simulink model "untitled1"  (R2023b)
settings: Solver=VariableStepAuto  StartTime=0.0  StopTime=10.0  RelTol=1e-3
libraries: dspsigops x1
settings Model: Creator=a2  LastModifiedBy=a2

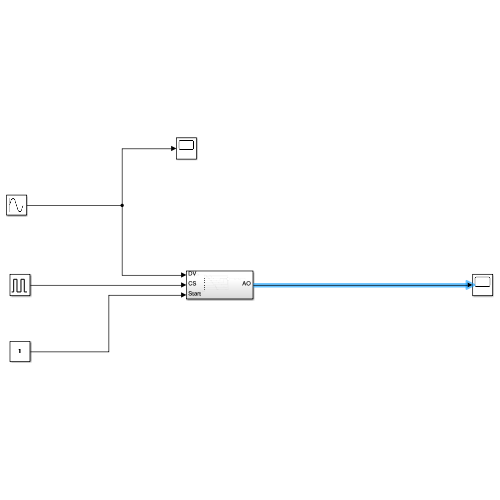
[thumbnail: Simulink's stored preview of the top-level diagram]
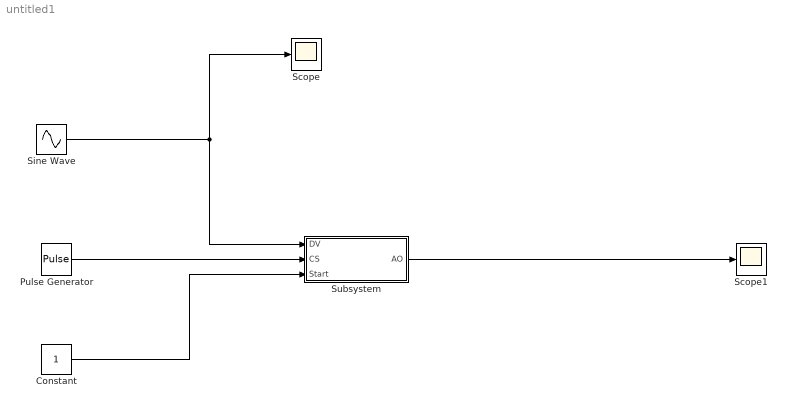
== system untitled1 ==
  Constant : Constant
  Pulse Generator : DiscretePulseGenerator  PulseType=Time based  Period=10  PulseWidth=5
  Scope : Scope
  Scope1 : Scope
  Sine Wave : Sin  SampleTime=0
  Subsystem : Subsystem
  wires:
  Sine Wave/1 -> Subsystem/1(DV), Scope/1
  Pulse Generator/1 -> Subsystem/2(CS)
  Constant/1 -> Subsystem/3(Start)
  Subsystem/1(AO) -> Scope1/1

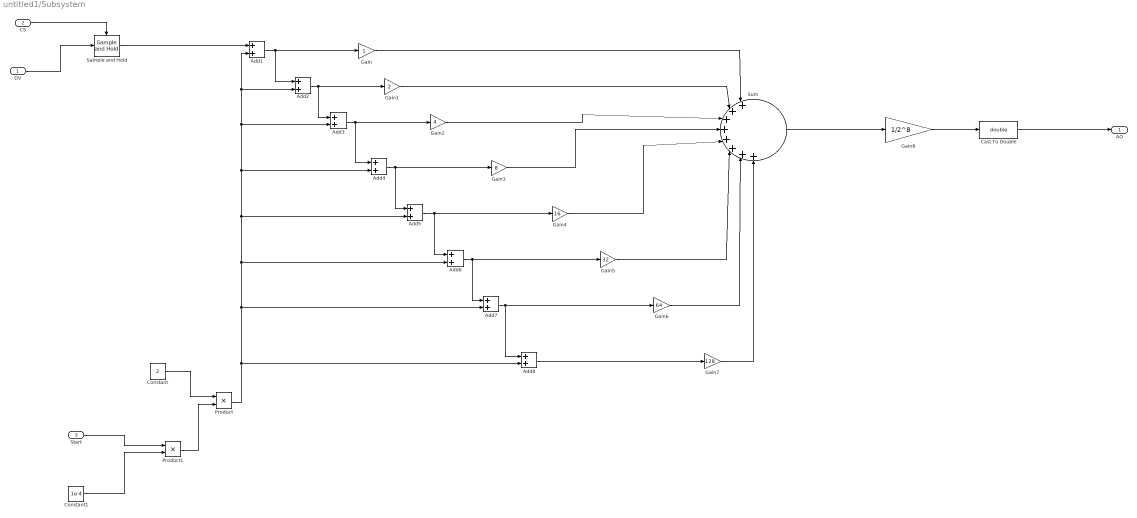
== system untitled1/Subsystem ==
  DV : Inport
  CS : Inport  Port=2
  Start : Inport  Port=3
  Add{1..8} (8 alike) : Sum
  Cast To Double : DataTypeConversion  OutDataTypeStr=double  SaturateOnIntegerOverflow=off  RndMeth=Floor
  Constant : Constant  Value=2
  Constant1 : Constant  Value=1e-4
  Gain : Gain
  Gain1 : Gain  Gain=2
  Gain2 : Gain  Gain=4
  Gain3 : Gain  Gain=8
  Gain4 : Gain  Gain=16
  Gain5 : Gain  Gain=32
  Gain6 : Gain  Gain=64
  Gain7 : Gain  Gain=128
  Gain8 : Gain  Gain=1/2^8
  Product : Product
  Product1 : Product
  Sample and Hold : dspsigops/Sample and Hold  trig=Rising edge  initCond=0  latchinput=off
  Sum : Sum  Inputs=|++++++++
  AO : Outport
  wires:
  CS/1 -> Sample and Hold/Trigger
  DV/1 -> Sample and Hold/1
  Add1/1 -> Add2/1, Gain/1
  Add2/1 -> Add3/1, Gain1/1
  Add3/1 -> Add4/1, Gain2/1
  Add4/1 -> Add5/1, Gain3/1
  Add5/1 -> Add6/1, Gain4/1
  Add6/1 -> Add7/1, Gain5/1
  Add7/1 -> Add8/1, Gain6/1
  Add8/1 -> Gain7/1
  Gain7/1 -> Sum/8
  Gain6/1 -> Sum/7
  Gain5/1 -> Sum/6
  Gain4/1 -> Sum/5
  Gain3/1 -> Sum/4
  Gain2/1 -> Sum/3
  Gain1/1 -> Sum/2
  Gain/1 -> Sum/1
  Sample and Hold/1 -> Add1/1
  Product/1 -> Add7/2, Add6/2, Add4/2, Add3/2, Add2/2, Add1/2, Add5/2, Add8/2
  Constant/1 -> Product/1
  Product1/1 -> Product/2
  Start/1 -> Product1/1
  Constant1/1 -> Product1/2
  Gain8/1 -> Cast To Double/1
  Sum/1 -> Gain8/1
  Cast To Double/1 -> AO/1
